simulink model "s_PID_final_SOPHIAUPEGUIR"  (R2022b)
settings: Solver=VariableStepAuto  StartTime=0.0  StopTime=2000  RelTol=1e-3
libraries: fuzblock x3, simulink x1
settings Model: Creator=sophy  LastModifiedBy=sophy

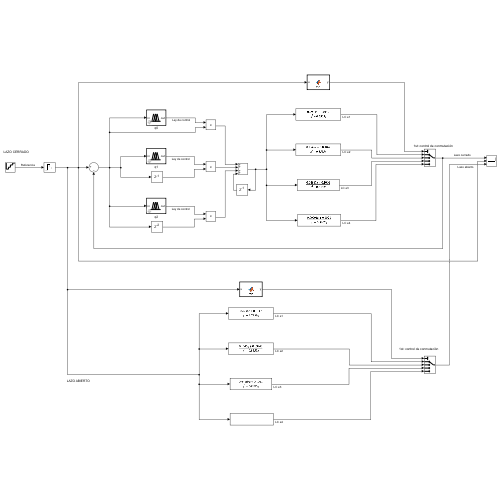
[thumbnail: Simulink's stored preview of the top-level diagram]
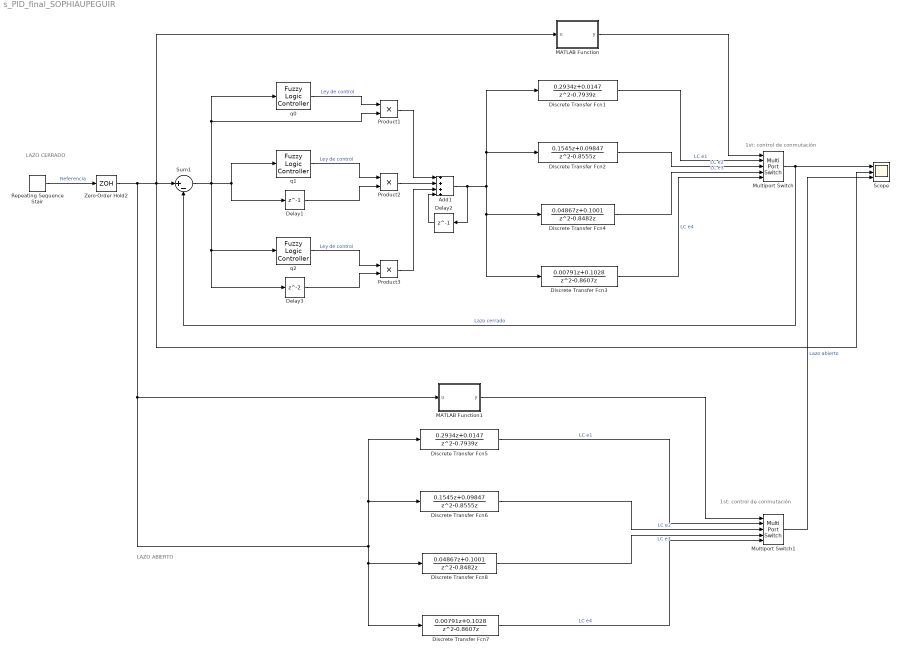
== system s_PID_final_SOPHIAUPEGUIR ==
  note: LAZO CERRADO
  note: 1st: control de conmutación
  note: 1st: control de conmutación
  note: LAZO ABIERTO
  Add1 : Sum  Inputs=++++
  Delay1 : Delay  DelayLength=1
  Delay2 : Delay  DelayLength=1
  Delay3 : Delay
  Discrete Transfer Fcn1 : DiscreteTransferFcn  Numerator=[0.2934 0.0147]  Denominator=[1 -0.7939 0]
  Discrete Transfer Fcn2 : DiscreteTransferFcn  Numerator=[0.1545 0.09847]  Denominator=[1 -0.8555 0]
  Discrete Transfer Fcn3 : DiscreteTransferFcn  Numerator=[0.00791 0.1028]  Denominator=[1 -0.8607 0]
  Discrete Transfer Fcn4 : DiscreteTransferFcn  Numerator=[0.04867 0.1001]  Denominator=[1 -0.8482 0]
  Discrete Transfer Fcn5 : DiscreteTransferFcn  Numerator=[0.2934 0.0147]  Denominator=[1 -0.7939 0]
  Discrete Transfer Fcn6 : DiscreteTransferFcn  Numerator=[0.1545 0.09847]  Denominator=[1 -0.8555 0]
  Discrete Transfer Fcn7 : DiscreteTransferFcn  Numerator=[0.00791 0.1028]  Denominator=[1 -0.8607 0]
  Discrete Transfer Fcn8 : DiscreteTransferFcn  Numerator=[0.04867 0.1001]  Denominator=[1 -0.8482 0]
  MATLAB Function : MATLAB Function  TreatAsAtomicUnit=on
  MATLAB Function1 : MATLAB Function  TreatAsAtomicUnit=on
  Multiport Switch : MultiPortSwitch  Inputs=4  SaturateOnIntegerOverflow=off  InputSameDT=off
  Multiport Switch1 : MultiPortSwitch  Inputs=4  SaturateOnIntegerOverflow=off  InputSameDT=off
  Product1 : Product
  Product2 : Product
  Product3 : Product
  Repeating Sequence Stair : simulink/Sources/Repeating Sequence Stair  OutValues=[20 30 40 50].'  tsamp=500  OutMin=[]  OutMax=[]  OutDataTypeStr=double  OutputDataTypeScalingMode=double  OutDataType=fixdt(0,8)  ConRadixGroup=Best Precision: Vector-wise  OutScaling=2^-12
  Scope : Scope  NumInputPorts=3
  Sum1 : Sum  Inputs=|+-
  Zero-Order Hold2 : ZeroOrderHold  SampleTime=7.5
  q0 : fuzblock/Fuzzy Logic  Controller  FIS=q0_e3  OutputSampleNumber=101  DataType=double  FuzzifiedInputs=off  RuleFiringStrengths=off  RuleOutputs=off  AggregatedOutputs=off  SimulateUsing=Interpreted execution  OutOfRangeInputValueMessage=warning  NoRuleFiredMessage=warning  EmptyOutputFuzzySetMessage=warning
  q1 : fuzblock/Fuzzy Logic  Controller  FIS=q1_e3  OutputSampleNumber=101  DataType=double  FuzzifiedInputs=off  RuleFiringStrengths=off  RuleOutputs=off  AggregatedOutputs=off  SimulateUsing=Interpreted execution  OutOfRangeInputValueMessage=warning  NoRuleFiredMessage=warning  EmptyOutputFuzzySetMessage=warning
  q2 : fuzblock/Fuzzy Logic  Controller  FIS=q2_e3  OutputSampleNumber=101  DataType=double  FuzzifiedInputs=off  RuleFiringStrengths=off  RuleOutputs=off  AggregatedOutputs=off  SimulateUsing=Interpreted execution  OutOfRangeInputValueMessage=warning  NoRuleFiredMessage=warning  EmptyOutputFuzzySetMessage=warning
  wires:
  Product2/1 -> Add1/2
  Repeating Sequence Stair/1 -> Zero-Order Hold2/1  "Referencia"
  Add1/1 -> Delay2/1, Discrete Transfer Fcn1/1, Discrete Transfer Fcn2/1, Discrete Transfer Fcn3/1, Discrete Transfer Fcn4/1
  Discrete Transfer Fcn4/1 -> Multiport Switch/4  "LC e3"
  Discrete Transfer Fcn1/1 -> Multiport Switch/2  "LC e1"
  MATLAB Function/1(y) -> Multiport Switch/1
  Discrete Transfer Fcn3/1 -> Multiport Switch/5  "LC e4"
  Discrete Transfer Fcn2/1 -> Multiport Switch/3  "LC e2"
  Product1/1 -> Add1/1
  Delay2/1 -> Add1/4
  Delay1/1 -> Product2/2
  Multiport Switch/1 -> Sum1/2, Scope/1  "Lazo cerrado"
  q0/1 -> Product1/1  "Ley de control"
  q1/1 -> Product2/1  "Ley de control"
  Discrete Transfer Fcn5/1 -> Multiport Switch1/2  "LC e1"
  Multiport Switch1/1 -> Scope/3  "Lazo abierto"
  Discrete Transfer Fcn6/1 -> Multiport Switch1/3  "LC e2"
  Zero-Order Hold2/1 -> Scope/2, MATLAB Function/1(u), Sum1/1, MATLAB Function1/1(u), Discrete Transfer Fcn5/1, Discrete Transfer Fcn6/1, Discrete Transfer Fcn7/1, Discrete Transfer Fcn8/1
  Discrete Transfer Fcn8/1 -> Multiport Switch1/4  "LC e3"
  Discrete Transfer Fcn7/1 -> Multiport Switch1/5  "LC e4"
  MATLAB Function1/1(y) -> Multiport Switch1/1
  Delay3/1 -> Product3/2
  q2/1 -> Product3/1  "Ley de control"
  Sum1/1 -> q2/1, Delay3/1, Delay1/1, q1/1, q0/1, Product1/2
  Product3/1 -> Add1/3

== matlab function s_PID_final_SOPHIAUPEGUIR/MATLAB Function ==
  data: u input; y output
function y = fcn(u)

if ((u>0)&&(u<=20)) % u = lo que entra = escalon
u = 1; % activar pin 1
end

if ((u>20)&&(u<=30))
u = 2; % activar pin 2
end 

if ((u>30)&&(u<=40))
u = 3; % activar pin 3
end 

if ((u>40)&&(u<=50))
u = 4; % activar pin 4
end 

y = u;

== matlab function s_PID_final_SOPHIAUPEGUIR/MATLAB Function1 ==
  data: u input; y output
function y = fcn(u)

if ((u>0)&&(u<=20)) % u = lo que entra = escalon
u = 1; % activar pin 1
end

if ((u>20)&&(u<=30))
u = 2; % activar pin 2
end 

if ((u>30)&&(u<=40))
u = 3; % activar pin 3
end 

if ((u>40)&&(u<=50))
u = 4; % activar pin 4
end 

y = u;
